simulink model "Bicycle_Model_RCVD_prev_version"  (R2022a)
settings: Solver=VariableStepAuto  StartTime=0.0  StopTime=60  RelTol=1e-3
values from neighbouring files (symbols this model uses):
  Battery_Voltage = 120    [RCVD.mat]
  CG_height = 0.6    [RCVD.mat]
  Cornering_Stiffness = 1000    [RCVD.mat]
  Gear_ratio = 6    [RCVD.mat]
  Mass = 250    [RCVD.mat]
  Max_Steer_Angle = 60    [RCVD.mat]
  Wheel_Base = 1.8    [RCVD.mat]
  Wheel_Radius = 0.211    [RCVD.mat]
  Width = 1    [RCVD.mat]
libraries: SignalEditorBlockLib x3, autolibmappedmotor x2
settings Model: Creator=User  LastModifiedBy=gautamd
settings ModelReferenceCC: EnableRefExpFcnMdlSchedulingChecks=off
settings RTWCC: Description=Generic Real-Time Target  GPUComputeCapability=5.0

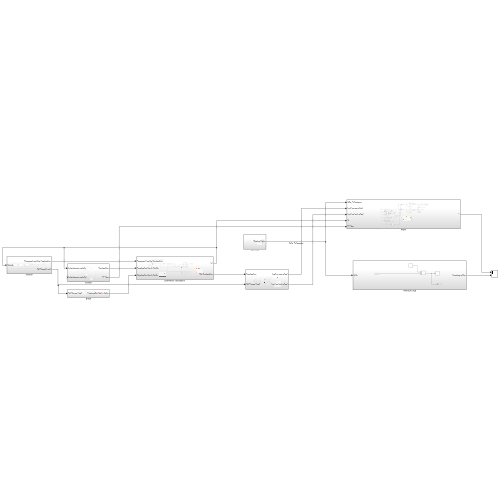
[thumbnail: Simulink's stored preview of the top-level diagram]
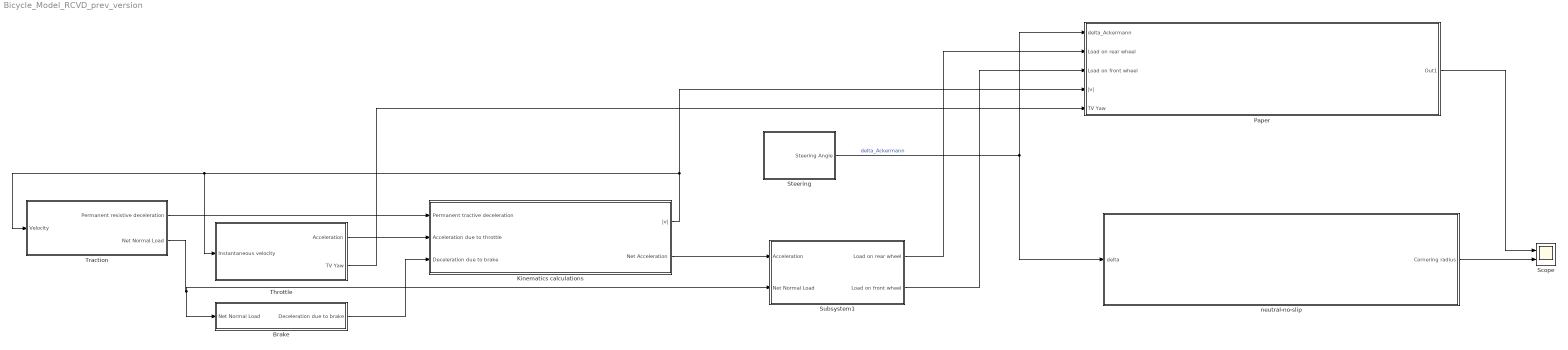
== system Bicycle_Model_RCVD_prev_version ==
  Brake : Subsystem
  Kinematics calculations : Subsystem
  Paper : Subsystem
  Scope : Scope  NumInputPorts=2
  Steering : Subsystem
  Subsystem1 : Subsystem
  Throttle : Subsystem
  Traction : Subsystem
  neutral-no-slip : Subsystem
  wires:
  Kinematics calculations/1(|v|) -> Traction/1(Velocity), Throttle/1(Instantaneous velocity), Paper/4(|v|)
  Steering/1(Steering Angle) -> neutral-no-slip/1(delta), Paper/1(delta_Ackermann)  "delta_Ackermann"
  Kinematics calculations/2(Net Acceleration) -> Subsystem1/1(Acceleration)
  Subsystem1/1(Load on rear wheel) -> Paper/2(Load on rear wheel)
  Subsystem1/2(Load on front wheel) -> Paper/3(Load on front wheel)
  neutral-no-slip/1(Cornering radius) -> Scope/2
  Throttle/1(Acceleration) -> Kinematics calculations/2(Acceleration due to throttle)
  Traction/2(Net Normal Load) -> Brake/1(Net Normal Load), Subsystem1/2(Net Normal Load)
  Traction/1(Permanent resistive deceleration) -> Kinematics calculations/1(Permanent tractive deceleration)
  Paper/1(Out1) -> Scope/1
  Throttle/2(TV Yaw) -> Paper/5(TV Yaw)
  Brake/1(Deceleration due to brake) -> Kinematics calculations/3(Deceleration due to brake)

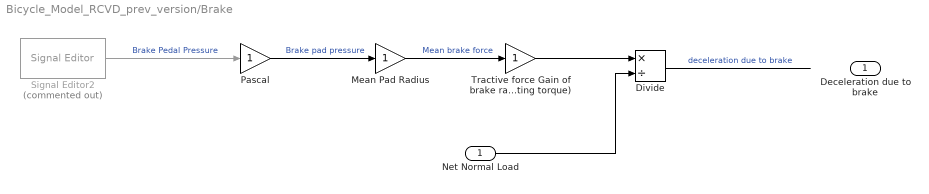
== system Bicycle_Model_RCVD_prev_version/Brake ==
  Net Normal Load : Inport
  Divide : Product  Inputs=*/
  Mean Pad Radius : Gain
  Pascal : Gain
  Signal Editor2 : SignalEditorBlockLib/Signal Editor  Commented=on  FileName=Brake_map.mat  ActiveScenario=Scenario  ActiveSignal=Signal 1  IsBus=off  OutputBusObjectStr=Bus: BusObject  SampleTime=0  Interpolate=off  ZeroCross=off  OutputAfterFinalValue=Setting to zero  Unit=inherit  PreserveSignalName=on
  Tractive force Gain of brake radius / wheel radius (equating torque) : Gain
  Deceleration due to brake : Outport
  wires:
  Signal Editor2/1 -> Pascal/1  "Brake Pedal Pressure"
  Pascal/1 -> Mean Pad Radius/1  "Brake pad pressure"
  Mean Pad Radius/1 -> Tractive force Gain of brake radius / wheel radius (equating torque)/1  "Mean brake force"
  Tractive force Gain of brake radius / wheel radius (equating torque)/1 -> Divide/1
  Divide/1 -> ?  "deceleration due to brake"
  Net Normal Load/1 -> Divide/2

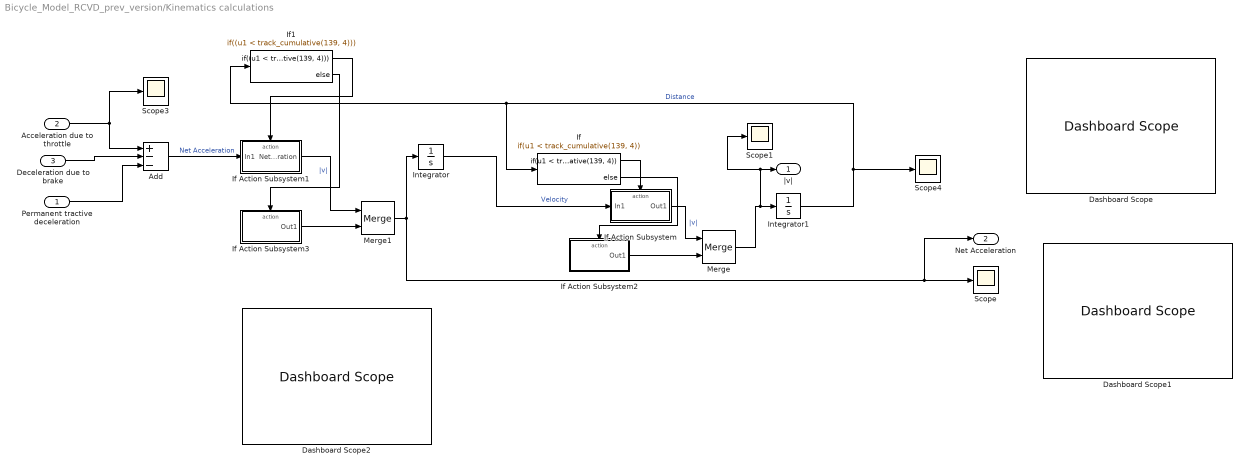
== system Bicycle_Model_RCVD_prev_version/Kinematics calculations ==
  Permanent tractive deceleration : Inport
  Acceleration due to throttle : Inport  Port=2
  Deceleration due to brake : Inport  Port=3
  Add : Sum  Inputs=+--
  Dashboard Scope : DashboardScope
  Dashboard Scope1 : DashboardScope
  Dashboard Scope2 : DashboardScope
  If : If  IfExpression=u1 < track_cumulative(139, 4)  ZeroCross=off
  If Action Subsystem : Subsystem  TreatAsAtomicUnit=on
  If Action Subsystem1 : Subsystem  TreatAsAtomicUnit=on
  If Action Subsystem2 : Subsystem  TreatAsAtomicUnit=on
  If Action Subsystem3 : Subsystem  TreatAsAtomicUnit=on
  If1 : If  IfExpression=(u1 < track_cumulative(139, 4))  ZeroCross=off
  Integrator : Integrator
  Integrator1 : Integrator
  Merge : Merge
  Merge1 : Merge
  Scope{,1,3..4} (4 alike) : Scope
  |v| : Outport
  Net Acceleration : Outport  Port=2
  wires:
  Integrator1/1 -> If1/1, If/1, Scope4/1  "Distance"
  Add/1 -> If Action Subsystem1/1(In1)  "Net Acceleration"
  If/1 -> If Action Subsystem/Action
  Integrator/1 -> If Action Subsystem/1(In1)  "Velocity"
  Permanent tractive deceleration/1 -> Add/3
  Acceleration due to throttle/1 -> Add/1, Scope3/1
  Deceleration due to brake/1 -> Add/2
  If1/1 -> If Action Subsystem1/Action
  If Action Subsystem1/1(Net Acceleration) -> Merge1/1  "|v|"
  If/2 -> If Action Subsystem2/Action
  If Action Subsystem2/1(Out1) -> Merge/2
  If Action Subsystem/1(Out1) -> Merge/1  "|v|"
  Merge/1 -> Scope1/1, |v|/1, Integrator1/1
  If Action Subsystem3/1(Out1) -> Merge1/2
  If1/2 -> If Action Subsystem3/Action
  Merge1/1 -> Integrator/1, Net Acceleration/1, Scope/1

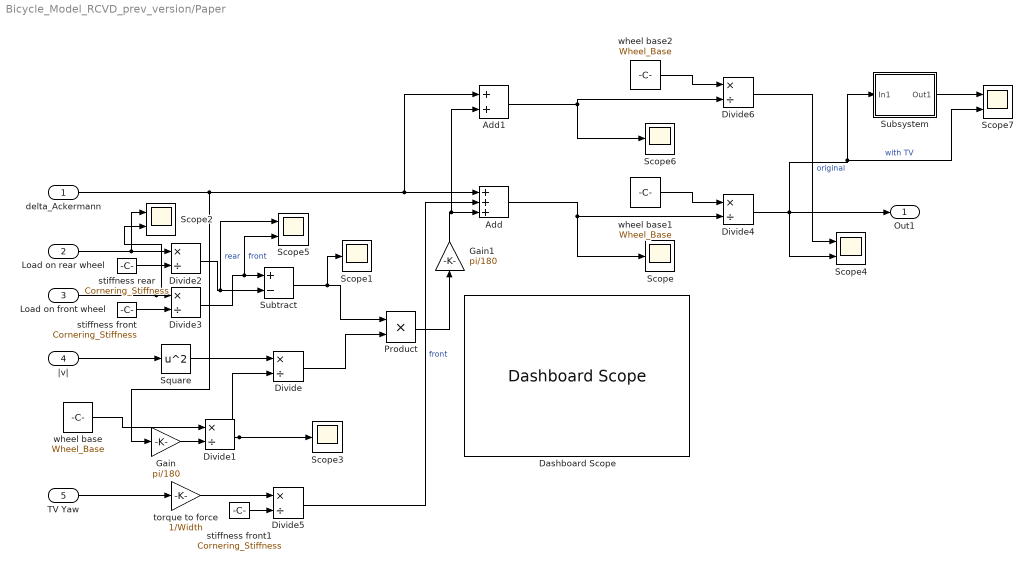
== system Bicycle_Model_RCVD_prev_version/Paper ==
  delta_Ackermann : Inport
  Load on rear wheel : Inport  Port=2
  Load on front wheel : Inport  Port=3
  |v| : Inport  Port=4
  TV Yaw : Inport  Port=5
  Add : Sum  Inputs=+++
  Add1 : Sum
  Dashboard Scope : DashboardScope
  Divide{,1..6} (7 alike) : Product  Inputs=*/
  Gain : Gain  Gain=pi/180
  Gain1 : Gain  Gain=pi/180
  Product : Product
  Scope{,1,3,6} (4 alike) : Scope
  Scope{2,4..5,7} (4 alike) : Scope  NumInputPorts=2
  Square : Math  Operator=square
  Subsystem : Subsystem
  Subtract : Sum  Inputs=+-
  stiffness front : Constant  Value=Cornering_Stiffness
  stiffness front1 : Constant  Value=Cornering_Stiffness
  stiffness rear : Constant  Value=Cornering_Stiffness
  torque to force : Gain  Gain=1/Width
  wheel base : Constant  Value=Wheel_Base
  wheel base1 : Constant  Value=Wheel_Base
  wheel base2 : Constant  Value=Wheel_Base
  Out1 : Outport
  wires:
  delta_Ackermann/1 -> Gain/1, Add1/1, Add/1
  |v|/1 -> Square/1
  Square/1 -> Divide/1
  wheel base/1 -> Divide1/1
  Divide1/1 -> Divide/2, Scope3/1
  Load on rear wheel/1 -> Scope2/1, Divide2/1
  Load on front wheel/1 -> Scope2/2, Divide3/1
  stiffness rear/1 -> Divide2/2
  stiffness front/1 -> Divide3/2
  Divide3/1 -> Scope5/2, Subtract/1  "front"
  Divide2/1 -> Subtract/2, Scope5/1  "rear"
  Subtract/1 -> Scope1/1, Product/1
  Divide/1 -> Product/2
  Product/1 -> Gain1/1
  Add/1 -> Divide4/2, Scope/1
  Gain/1 -> Divide1/2
  Divide4/1 -> Scope7/2, Subsystem/1(In1), Scope4/2, Out1/1  "with TV"
  wheel base1/1 -> Divide4/1
  Gain1/1 -> Add1/2, Add/3
  TV Yaw/1 -> torque to force/1
  torque to force/1 -> Divide5/1
  stiffness front1/1 -> Divide5/2
  Divide5/1 -> Add/2  "front"
  wheel base2/1 -> Divide6/1
  Add1/1 -> Divide6/2, Scope6/1
  Divide6/1 -> Scope4/1  "original"
  Subsystem/1(Out1) -> Scope7/1

== system Bicycle_Model_RCVD_prev_version/Steering ==
  10 : Constant  Value=10
  Dashboard Scope : DashboardScope
  MATLAB Function : MATLAB Function  TreatAsAtomicUnit=on
  Max_Steer_Angle : Constant  Value=Max_Steer_Angle
  Scope : Scope
  Steering Angle : Outport
  wires:
  MATLAB Function/1(y) -> Scope/1, Steering Angle/1
  Max_Steer_Angle/1 -> MATLAB Function/2(Max_Steer_Angle)
  10/1 -> MATLAB Function/1(u)

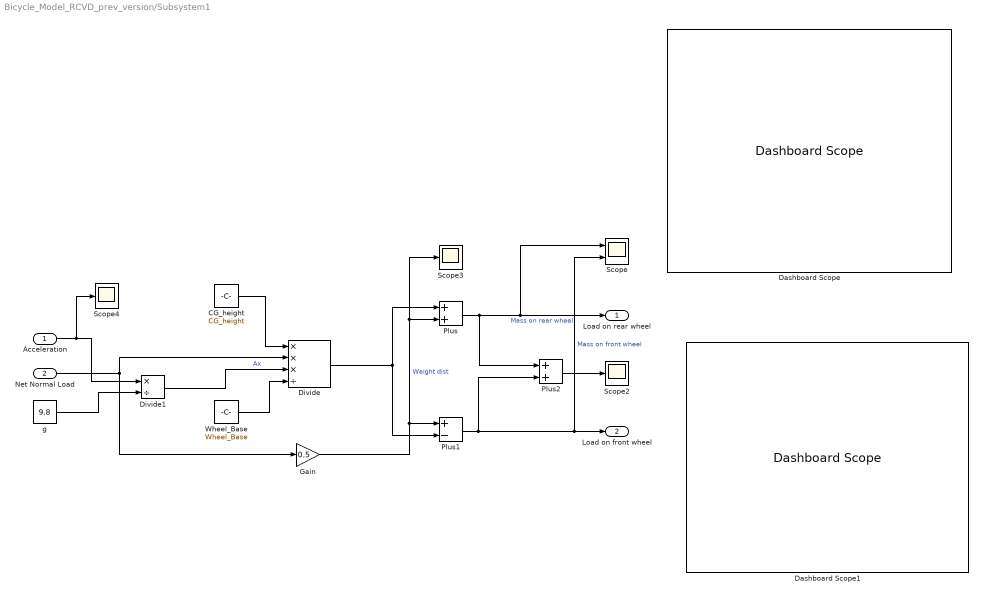
== system Bicycle_Model_RCVD_prev_version/Subsystem1 ==
  Acceleration : Inport
  Net Normal Load : Inport  Port=2
  CG_height : Constant  Value=CG_height
  Dashboard Scope : DashboardScope
  Dashboard Scope1 : DashboardScope
  Divide : Product  Inputs=***/
  Divide1 : Product  Inputs=*/
  Gain : Gain  Gain=0.5
  Plus : Sum
  Plus1 : Sum  Inputs=+-
  Plus2 : Sum
  Scope : Scope  NumInputPorts=2
  Scope2 : Scope
  Scope3 : Scope
  Scope4 : Scope
  Wheel_Base : Constant  Value=Wheel_Base
  g : Constant  Value=9.8
  Load on rear wheel : Outport
  Load on front wheel : Outport  Port=2
  wires:
  g/1 -> Divide1/2
  Divide/1 -> Plus1/2, Plus/1
  Acceleration/1 -> Scope4/1, Divide1/1
  Gain/1 -> Scope3/1, Plus/2, Plus1/1  "Weight dist"
  CG_height/1 -> Divide/1
  Wheel_Base/1 -> Divide/4
  Divide1/1 -> Divide/3  "Ax"
  Plus/1 -> Scope/1, Load on rear wheel/1, Plus2/1  "Mass on rear wheel"
  Plus1/1 -> Scope/2, Load on front wheel/1, Plus2/2  "Mass on front wheel"
  Net Normal Load/1 -> Divide/2, Gain/1
  Plus2/1 -> Scope2/1

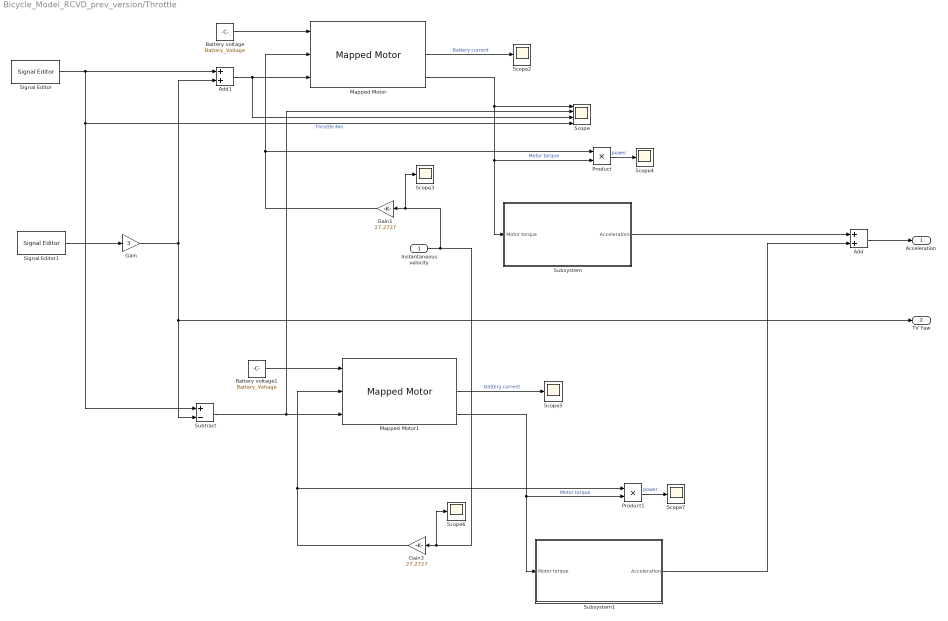
== system Bicycle_Model_RCVD_prev_version/Throttle ==
  Instantaneous velocity : Inport
  Add : Sum
  Add1 : Sum
  Battery voltage : Constant  Value=Battery_Voltage
  Battery voltage1 : Constant  Value=Battery_Voltage
  Gain : Gain  Gain=3
  Gain1 : Gain  Gain=27.2727
  Gain3 : Gain  Gain=27.2727
  Mapped Motor : autolibmappedmotor/Mapped Motor  port_config=Speed  param_by=Maximum torque and power  w_t=[ 0 375 750 800 ]  T_t=[0.09 0.08 0.07 0]  torque_max=29  power_max=Max_Power  Tc=0.1  param_loss=Single efficiency measurement  eff=93  w_eff=600  T_eff=29  Piron=0  Pbase=0  w_eff_bp=[-8000 -4000 0 4000 8000]  T_eff_bp=[0 0.03 0.06 0.09]  Temp_eff_bp=[233.15 293.15 373.15]  losses_table=[1.49 1.67 2.21 3.10; 0.42 0.69 1.14 2.03; 0.06 0.24 0.78 1.68; 0.42 0.69 1.14 2.03; 1.49 1.67 2.21 3.10]  losses_table_3d=cat(3,1.05*[1.49 1.67 2.21 3.10; 0.42 0.69 1.14 2.03; 0.06 0.24 0.78 1.68; 0.42 0.69 1.14 2.03; 1.49 1.67 2.21 3.10],[1.49 1.67 2.21 3.10; 0.42 0.69 1.14 2.03; 0.06 0.24 0.78 1.68; 0.42 0.69 1.14 2.03; 1.49 1.67 2.21 3.10],1.03*[1.49 1.67 2.21 3.10; 0.42 0.69 1.14 2.03; 0.06 0.24 0.78 1.68; 0.42 0.69 1.14 2.03; 1.49 1.67 2.21 3.10])  efficiency_table=[95 95 95 95; 95 95 95 95; 95 95 95 95; 95 95 95 95; 95 95 95 95]  efficiency_table_3d=cat(3,90*ones(5,4),95*ones(5,4),92*ones(5,4))  J=0.021  b=1e-5  omega_o=0  T_t_extended=[0 0.07 0.08 0.09 0.08 0.07 0]  w_t_extended=[-800 -750 -375 0 375 750 800]  KLossIron=0  KLossCopper=1.5573  x_w_eff_vec=[-8000 -4000 0 4000 8000]  x_T_eff_vec=[-0.09 -0.06 -0.03 0 0.03 0.06 0.09]  x_tmp_eff_vec=[233.15 293.15 373.15]  x_losses_mat=[3.1 2.21 1.67 1.49 1.67 2.21 3.1;2.03 1.14 0.69 0.42 0.69 1.14 2.03;1.68 0.78 0.24 0.06 0.24 0.78 1.68;2.03 1.14 0.69 0.42 0.69 1.14 2.03;3.1 2.21 1.67 1.49 1.67 2.21 3.1]  x_losses_mat_3d=cat(3,[3.255 2.3205 1.7535 1.5645 1.7535 2.3205 3.255;2.1315 1.197 0.7245 0.441 0.7245 1.197 2.1315;1.764 0.819 0.252 0.063 0.252 0.819 1.764;2.1315 1.197 0.7245 0.441 0.7245 1.197 2.1315;3.255 2.3205 1.7535 1.5645 1.7535 2.3205 3.255],[3.1 2.21 1.67 1.49 1.67 2.21 3.1;2.03 1.14 0.69 0.42 0.69 1.14 2.03;1.68 0.78 0.24 0.06 0.24 0.78 1.68;2.03 1.14 0.69 0.42 0.69 1.14 2.03;3.1 2.21 1.67 1.49 1.67 2.21 3.1],[3.193 2.2763 1.7201 1.5347 1.7201 2.2763 3.193;2.0909 1.1742 0.7107 0.4326 0.7107 1.1742 2.0909;1.7304 0.8034 0.2472 0.0618 0.2472 0.8034 1.7304;2.0909 1.1742 0.7107 0.4326 0.7107 1.1742 2.0909;3.193 2.2763 1.7201 1.5347 1.7201 2.2763 3.193])  CalLossMapData={}  CalLossWithTempMapData={}  aMode=2  RefBlkName='autolibmappedmotor/Mapped Motor'
      settings: SourceProductBaseCode=PW,DR,MT,VE
  Mapped Motor1 : autolibmappedmotor/Mapped Motor  port_config=Speed  param_by=Maximum torque and power  w_t=[ 0 375 750 800 ]  T_t=[0.09 0.08 0.07 0]  torque_max=29  power_max=Max_Power  Tc=0.1  param_loss=Single efficiency measurement  eff=93  w_eff=600  T_eff=29  Piron=0  Pbase=0  w_eff_bp=[-8000 -4000 0 4000 8000]  T_eff_bp=[0 0.03 0.06 0.09]  Temp_eff_bp=[233.15 293.15 373.15]  losses_table=[1.49 1.67 2.21 3.10; 0.42 0.69 1.14 2.03; 0.06 0.24 0.78 1.68; 0.42 0.69 1.14 2.03; 1.49 1.67 2.21 3.10]  losses_table_3d=cat(3,1.05*[1.49 1.67 2.21 3.10; 0.42 0.69 1.14 2.03; 0.06 0.24 0.78 1.68; 0.42 0.69 1.14 2.03; 1.49 1.67 2.21 3.10],[1.49 1.67 2.21 3.10; 0.42 0.69 1.14 2.03; 0.06 0.24 0.78 1.68; 0.42 0.69 1.14 2.03; 1.49 1.67 2.21 3.10],1.03*[1.49 1.67 2.21 3.10; 0.42 0.69 1.14 2.03; 0.06 0.24 0.78 1.68; 0.42 0.69 1.14 2.03; 1.49 1.67 2.21 3.10])  efficiency_table=[95 95 95 95; 95 95 95 95; 95 95 95 95; 95 95 95 95; 95 95 95 95]  efficiency_table_3d=cat(3,90*ones(5,4),95*ones(5,4),92*ones(5,4))  J=0.021  b=1e-5  omega_o=0  T_t_extended=[0 0.07 0.08 0.09 0.08 0.07 0]  w_t_extended=[-800 -750 -375 0 375 750 800]  KLossIron=0  KLossCopper=1.5573  x_w_eff_vec=[-8000 -4000 0 4000 8000]  x_T_eff_vec=[-0.09 -0.06 -0.03 0 0.03 0.06 0.09]  x_tmp_eff_vec=[233.15 293.15 373.15]  x_losses_mat=[3.1 2.21 1.67 1.49 1.67 2.21 3.1;2.03 1.14 0.69 0.42 0.69 1.14 2.03;1.68 0.78 0.24 0.06 0.24 0.78 1.68;2.03 1.14 0.69 0.42 0.69 1.14 2.03;3.1 2.21 1.67 1.49 1.67 2.21 3.1]  x_losses_mat_3d=cat(3,[3.255 2.3205 1.7535 1.5645 1.7535 2.3205 3.255;2.1315 1.197 0.7245 0.441 0.7245 1.197 2.1315;1.764 0.819 0.252 0.063 0.252 0.819 1.764;2.1315 1.197 0.7245 0.441 0.7245 1.197 2.1315;3.255 2.3205 1.7535 1.5645 1.7535 2.3205 3.255],[3.1 2.21 1.67 1.49 1.67 2.21 3.1;2.03 1.14 0.69 0.42 0.69 1.14 2.03;1.68 0.78 0.24 0.06 0.24 0.78 1.68;2.03 1.14 0.69 0.42 0.69 1.14 2.03;3.1 2.21 1.67 1.49 1.67 2.21 3.1],[3.193 2.2763 1.7201 1.5347 1.7201 2.2763 3.193;2.0909 1.1742 0.7107 0.4326 0.7107 1.1742 2.0909;1.7304 0.8034 0.2472 0.0618 0.2472 0.8034 1.7304;2.0909 1.1742 0.7107 0.4326 0.7107 1.1742 2.0909;3.193 2.2763 1.7201 1.5347 1.7201 2.2763 3.193])  CalLossMapData={}  CalLossWithTempMapData={}  aMode=2  RefBlkName='autolibmappedmotor/Mapped Motor'
      settings: SourceProductBaseCode=PW,DR,MT,VE
  Product : Product
  Product1 : Product
  Scope : Scope  NumInputPorts=4
  Scope{2..7} (6 alike) : Scope
  Signal Editor : SignalEditorBlockLib/Signal Editor  FileName=Throttle_map.mat  ActiveScenario=Scenario  ActiveSignal=Signal 1  IsBus=off  OutputBusObjectStr=Bus: BusObject  SampleTime=0  Interpolate=off  ZeroCross=off  OutputAfterFinalValue=Setting to zero  Unit=inherit  PreserveSignalName=on
  Signal Editor1 : SignalEditorBlockLib/Signal Editor  FileName=Torque vectoring input.mat  ActiveScenario=Scenario  ActiveSignal=Signal 1  IsBus=off  OutputBusObjectStr=Bus: BusObject  SampleTime=0  Interpolate=off  ZeroCross=off  OutputAfterFinalValue=Setting to zero  Unit=inherit  PreserveSignalName=on
  Subsystem : Subsystem
  Subsystem1 : Subsystem
  Subtract : Sum  Inputs=+-
  Acceleration : Outport
  TV Yaw : Outport  Port=2
  wires:
  Battery voltage/1 -> Mapped Motor/1
  Signal Editor/1 -> Scope/4, Subtract/1, Add1/1  "Throttle Nm"
  Mapped Motor/2 -> Scope2/1  "Battery current"
  Mapped Motor/3 -> Product/2, Subsystem/1(Motor torque), Scope/1  "Motor torque"
  Gain1/1 -> Product/1, Mapped Motor/2
  Product/1 -> Scope4/1  "power"
  Subsystem1/1(Acceleration) -> Add/2
  Product1/1 -> Scope7/1  "power"
  Mapped Motor1/2 -> Scope5/1  "Battery current"
  Mapped Motor1/3 -> Product1/2, Subsystem1/1(Motor torque)  "Motor torque"
  Instantaneous velocity/1 -> Scope6/1, Gain3/1, Scope3/1, Gain1/1
  Gain3/1 -> Product1/1, Mapped Motor1/2
  Battery voltage1/1 -> Mapped Motor1/1
  Add/1 -> Acceleration/1
  Subsystem/1(Acceleration) -> Add/1
  Signal Editor1/1 -> Gain/1
  Add1/1 -> Scope/3, Mapped Motor/3
  Subtract/1 -> Scope/2, Mapped Motor1/3
  Gain/1 -> Add1/2, TV Yaw/1, Subtract/2

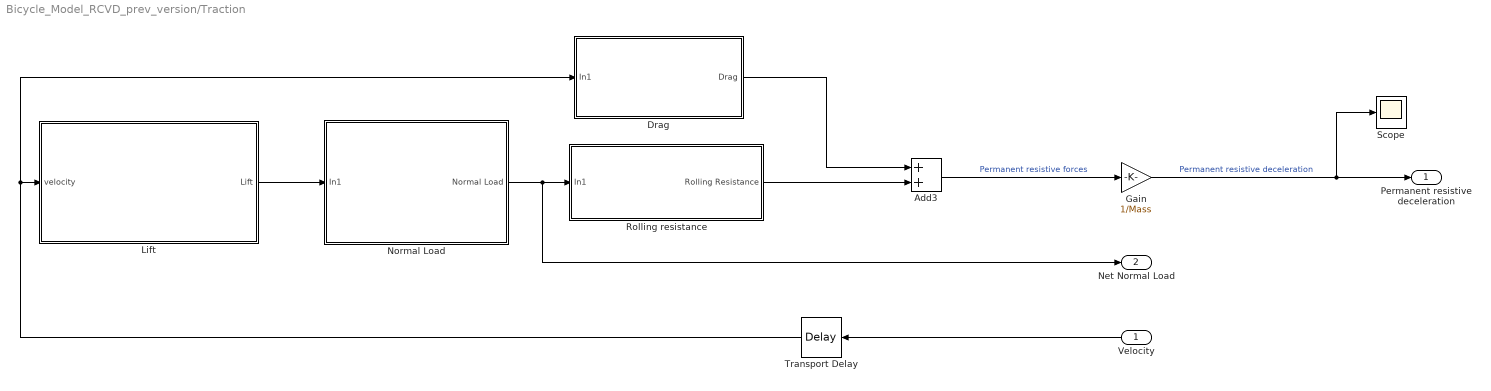
== system Bicycle_Model_RCVD_prev_version/Traction ==
  Velocity : Inport
  Add3 : Sum
  Drag : Subsystem
  Gain : Gain  Gain=1/Mass
  Lift : Subsystem
  Normal Load : Subsystem
  Rolling resistance : Subsystem
  Scope : Scope
  Transport Delay : TransportDelay  DelayTime=0.1
  Permanent resistive deceleration : Outport
  Net Normal Load : Outport  Port=2
  wires:
  Velocity/1 -> Transport Delay/1
  Lift/1(Lift) -> Normal Load/1(In1)
  Rolling resistance/1(Rolling Resistance) -> Add3/2
  Transport Delay/1 -> Drag/1(In1), Lift/1(velocity)
  Normal Load/1(Normal Load) -> Net Normal Load/1, Rolling resistance/1(In1)
  Drag/1(Drag) -> Add3/1
  Gain/1 -> Scope/1, Permanent resistive deceleration/1  "Permanent resistive deceleration"
  Add3/1 -> Gain/1  "Permanent resistive forces"

== system Bicycle_Model_RCVD_prev_version/neutral-no-slip ==
  delta : Inport
  Divide1 : Product  Inputs=*/
  Scope7 : Scope
  Wheel Base : Constant  Value=Wheel_Base
  Cornering radius : Outport
  wires:
  Wheel Base/1 -> Divide1/1
  Divide1/1 -> Cornering radius/1, Scope7/1  "R"
  delta/1 -> Divide1/2  "net delta"

== system Bicycle_Model_RCVD_prev_version/Kinematics calculations/If Action Subsystem ==
  In1 : Inport
  Action Port : ActionPort  ActionPortLabel=if(u1 < track_cumulative(139, 4))
  Gain : Gain
  Out1 : Outport
  wires:
  In1/1 -> Gain/1
  Gain/1 -> Out1/1

== system Bicycle_Model_RCVD_prev_version/Kinematics calculations/If Action Subsystem1 ==
  In1 : Inport
  Action Port : ActionPort  ActionPortLabel=if((u1 < track_cumulative(139, 4)))
  Gain : Gain
  Net Acceleration : Outport
  wires:
  In1/1 -> Gain/1
  Gain/1 -> Net Acceleration/1

== system Bicycle_Model_RCVD_prev_version/Kinematics calculations/If Action Subsystem2 ==
  Action Port : ActionPort  ActionPortLabel=else
  Constant : Constant  Value=0
  Out1 : Outport
  wires:
  Constant/1 -> Out1/1

== system Bicycle_Model_RCVD_prev_version/Kinematics calculations/If Action Subsystem3 ==
  Action Port : ActionPort  ActionPortLabel=else
  Constant : Constant  Value=0
  Out1 : Outport
  wires:
  Constant/1 -> Out1/1

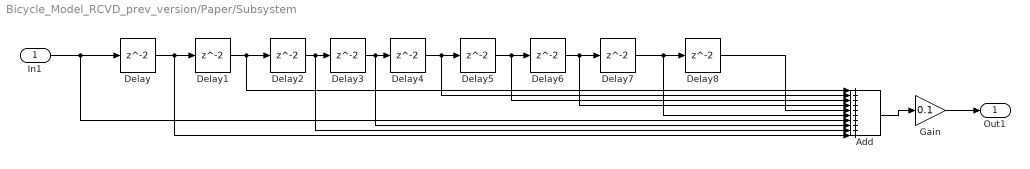
== system Bicycle_Model_RCVD_prev_version/Paper/Subsystem ==
  In1 : Inport
  Add : Sum  Inputs=++++++++++
  Delay : Delay  SampleTime=0.01
  Delay{1..8} (8 alike) : Delay
  Gain : Gain  Gain=0.1
  Out1 : Outport
  wires:
  Delay/1 -> Add/10, Delay1/1
  In1/1 -> Add/7, Delay/1
  Delay1/1 -> Add/1, Delay2/1
  Delay2/1 -> Add/9, Delay3/1
  Delay3/1 -> Add/8, Delay4/1
  Delay4/1 -> Add/2, Delay5/1
  Delay5/1 -> Add/3, Delay6/1
  Delay6/1 -> Add/4, Delay7/1
  Add/1 -> Gain/1
  Delay7/1 -> Delay8/1, Add/6
  Gain/1 -> Out1/1
  Delay8/1 -> Add/5

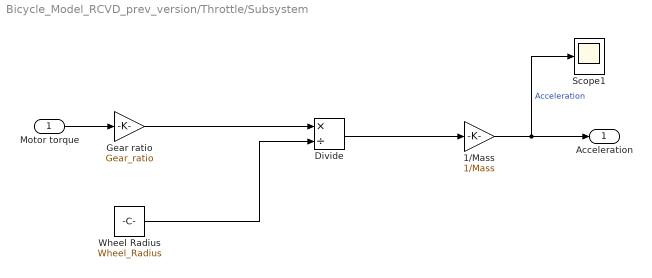
== system Bicycle_Model_RCVD_prev_version/Throttle/Subsystem ==
  Motor torque : Inport
  1/Mass : Gain  Gain=1/Mass
  Divide : Product  Inputs=*/
  Gear ratio : Gain  Gain=Gear_ratio
  Scope1 : Scope
  Wheel Radius : Constant  Value=Wheel_Radius
  Acceleration : Outport
  wires:
  Divide/1 -> 1/Mass/1
  Gear ratio/1 -> Divide/1
  Wheel Radius/1 -> Divide/2
  1/Mass/1 -> Acceleration/1, Scope1/1  "Acceleration"
  Motor torque/1 -> Gear ratio/1

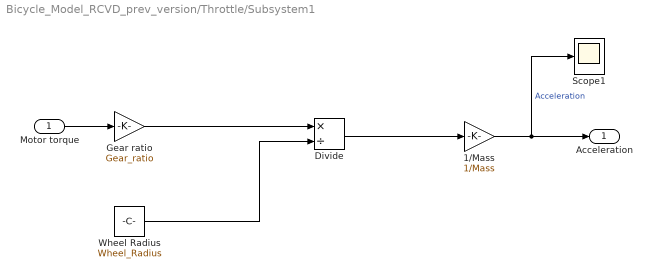
== system Bicycle_Model_RCVD_prev_version/Throttle/Subsystem1 ==
  Motor torque : Inport
  1/Mass : Gain  Gain=1/Mass
  Divide : Product  Inputs=*/
  Gear ratio : Gain  Gain=Gear_ratio
  Scope1 : Scope
  Wheel Radius : Constant  Value=Wheel_Radius
  Acceleration : Outport
  wires:
  Divide/1 -> 1/Mass/1
  Gear ratio/1 -> Divide/1
  Wheel Radius/1 -> Divide/2
  1/Mass/1 -> Acceleration/1, Scope1/1  "Acceleration"
  Motor torque/1 -> Gear ratio/1

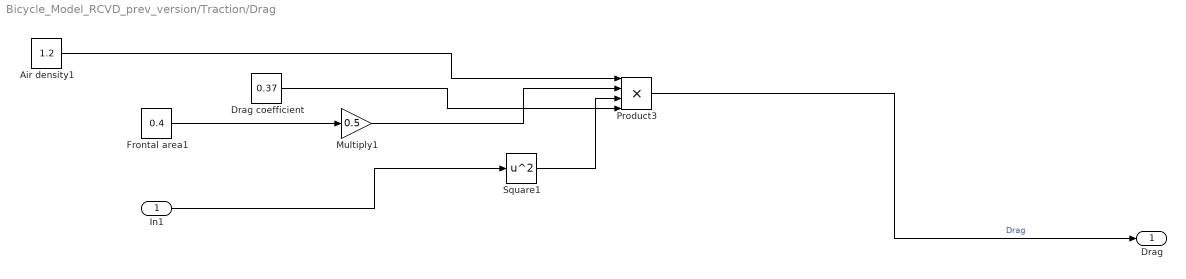
== system Bicycle_Model_RCVD_prev_version/Traction/Drag ==
  In1 : Inport
  Air density1 : Constant  Value=1.2
  Drag coefficient : Constant  Value=0.37
  Frontal area1 : Constant  Value=0.4
  Multiply1 : Gain  Gain=0.5
  Product3 : Product  Inputs=4
  Square1 : Math  Operator=square
  Drag : Outport
  wires:
  Multiply1/1 -> Product3/2
  Square1/1 -> Product3/3
  In1/1 -> Square1/1
  Air density1/1 -> Product3/1
  Frontal area1/1 -> Multiply1/1
  Drag coefficient/1 -> Product3/4
  Product3/1 -> Drag/1  "Drag"

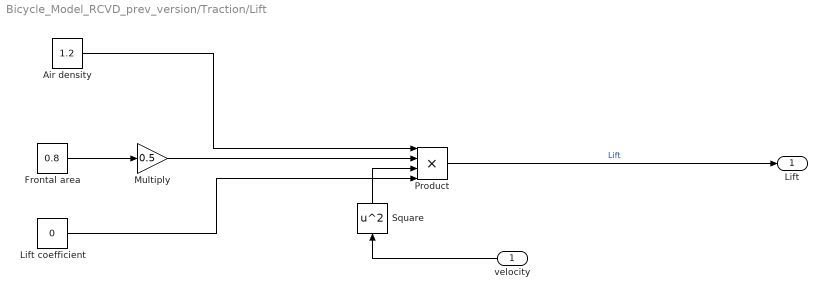
== system Bicycle_Model_RCVD_prev_version/Traction/Lift ==
  velocity : Inport
  Air density : Constant  Value=1.2
  Frontal area : Constant  Value=0.8
  Lift coefficient : Constant  Value=0
  Multiply : Gain  Gain=0.5
  Product : Product  Inputs=4
  Square : Math  Operator=square
  Lift : Outport
  wires:
  Frontal area/1 -> Multiply/1
  Multiply/1 -> Product/2
  Lift coefficient/1 -> Product/4
  Air density/1 -> Product/1
  Square/1 -> Product/3
  velocity/1 -> Square/1
  Product/1 -> Lift/1  "Lift"

== system Bicycle_Model_RCVD_prev_version/Traction/Normal Load ==
  In1 : Inport
  Add1 : Sum  Inputs=+-
  Mass : Constant  Value=Mass
  Product1 : Product
  g : Constant  Value=9.8
  Normal Load : Outport
  wires:
  g/1 -> Product1/1
  Product1/1 -> Add1/1  "Car weight"
  Mass/1 -> Product1/2
  Add1/1 -> Normal Load/1  "Normal Load"
  In1/1 -> Add1/2

== system Bicycle_Model_RCVD_prev_version/Traction/Rolling resistance ==
  In1 : Inport
  Product5 : Product
  Rolling resistance coefficient : Constant  Value=0
  Rolling Resistance : Outport
  wires:
  Rolling resistance coefficient/1 -> Product5/1
  Product5/1 -> Rolling Resistance/1  "Rolling Resistance"
  In1/1 -> Product5/2

== matlab function Bicycle_Model_RCVD_prev_version/Steering/MATLAB Function ==
  data: u input; y output; Max_Steer_Angle input
function y = fcn(u, Max_Steer_Angle)

y = u*Max_Steer_Angle*pi/18000;
